simulink model "v2022_Modello_SITL_AENEA_2020b"  (R2020b)
settings: Solver=ode4  StartTime=0.0  StopTime=500  FixedStep=0.01  RelTol=1e-3
values from neighbouring files (symbols this model uses):
  attuatore_Amax = 20*(pi/180)    (= 0.349065850399)    [v2021_10_27_avvioSITL.m]
  attuatore_Emax = 25*(pi/180)    (= 0.436332312999)    [v2021_10_27_avvioSITL.m]
  attuatore_Rmax = 25*(pi/180)    (= 0.436332312999)    [v2021_10_27_avvioSITL.m]
  beta_phi = 1/10.5600    (= 0.094696969697)    [Load_modello_sensori.m]
  beta_psi = 1/170    (= 0.00588235294118)    [Load_modello_sensori.m]
  beta_theta = 1/10.5000    (= 0.0952380952381)    [Load_modello_sensori.m]
  CldR = KCldR(1)*180/pi    [Timone.m]
  CndR = KCndR(1)*180/pi    [Timone.m]
  CYdR = -KCYdR(1)*180/pi    [Timone.m]
  delay_ahrs = 0    [Load_modello_sensori.m]
  delay_bmp = 0    [Load_modello_sensori.m]
  delay_gps = 0    [Load_modello_sensori.m]
  deltaAtrim = 0    [v2021_10_27_avvioSITL.m]
  deltaEtrim = (Cm0*CL_alpharad+Cm_alpharad*CLtrim)/(CL_alpharad*CmdE)    [calcoloDatiIniziali.m]    (also in v2021_10_27_avvioSITL.m = 0)
  deltaRtrim = 0    [v2021_10_27_avvioSITL.m]
  deltaTtrim = 0.1    [v2021_10_27_avvioSITL.m]
  HINI = -State0.Pos0(3)    [v2021_10_27_avvioSITL.m]
  Ingaggio_AP = input("inserire 1 se si vuole ingaggiare l' AP, 0 altrimenti: ")    [v2021_10_27_avvioSITL.m]
  J_vec = [0 0.03 0.06 0.09 0.11 0.14 0.17 0.2 0.23 0.26 0.28 0.31 ... (30 elements, 30x1)]    [PropLUT.mat]
  latitudineINI = 42.07278258649732*pi/180    (= 0.73430858161)    [v2021_10_27_avvioSITL.m]
  longitudineINI = 12.615743929793046*pi/180    (= 0.220186269163)    [v2021_10_27_avvioSITL.m]
  mean_ax = 0*0.0392    (= 0)    [Load_modello_sensori.m]
  mean_ay = -0*0.0598    (= 0)    [Load_modello_sensori.m]
  mean_az = 0*0.0384    (= 0)    [Load_modello_sensori.m]
  mean_p = 0*1.5184e-06    (= 0)    [Load_modello_sensori.m]
  mean_q = 0*2.9671e-05    (= 0)    [Load_modello_sensori.m]
  mean_r = 0*5.4105e-05    (= 0)    [Load_modello_sensori.m]
  P_ref = 1.0074e+05    (= 100740)    [Load_modello_sensori.m]
  PWM_Aileron = rad2deg(deltaAtrim)*9+1503    [v2021_10_27_avvioSITL.m]
  PWM_Elevator = rad2deg(deltaEtrim)*(447/50)+(3007/2)    [v2021_10_27_avvioSITL.m]
  PWM_Rudder = rad2deg(deltaRtrim)*(447/50)+(3007/2)    [v2021_10_27_avvioSITL.m]
  PWM_Throttle = (deltaTtrim)*800+1100    (= 1180)    [v2021_10_27_avvioSITL.m]
  seed_ahrs = randi([0 2000],1,1)    [Load_modello_sensori.m]
  seed_baro = randi([0 2000],1,1)    [Load_modello_sensori.m]
  seed_gps = randi([0 2000],1,1)    [Load_modello_sensori.m]
  sensori_FreqCampionamento_pitot = 0.02    [v2021_10_27_avvioSITL.m]
  sensori_RumoreSampleTime = 0.02    [v2021_10_27_avvioSITL.m]
  sensori_varianza = 0.0000    (= 0)    [v2021_10_27_avvioSITL.m]
  Std_con_lat = 7.501025208540287e-07    (= 7.50102520854e-07)    [Load_modello_sensori.m]
  Std_con_long = 5.101110498551838e-06    (= 5.10111049855e-06)    [Load_modello_sensori.m]
  Std_vel = 0.05    [Load_modello_sensori.m]
  T0_ref = 25    [Load_modello_sensori.m]
  Ta_lat = 10^2    (= 100)    [Load_modello_sensori.m]
  Ta_long = 10^2    (= 100)    [Load_modello_sensori.m]
  Ts_ahrs = 0.02    [Load_modello_sensori.m]
  Ts_bmp = 0.02    [Load_modello_sensori.m]
  Ts_gps = 0.1    [Load_modello_sensori.m]
  tsamp = 0.02    [v2021_10_27_avvioSITL.m]
  Var_heading = 0.0025    [Load_modello_sensori.m]
  Var_heading_static = 0.0625    [Load_modello_sensori.m]
  Var_V_hor = 0.1    [Load_modello_sensori.m]
  Var_V_hor_static = 0.04    [Load_modello_sensori.m]
  White_ax = 1.486e-04    (= 0.0001486)    [Load_modello_sensori.m]
  White_ay = 9.403e-05    [Load_modello_sensori.m]
  White_az = 1.648e-04    (= 0.0001648)    [Load_modello_sensori.m]
  White_gm_phi = 3.2740e-05    (= 3.274e-05)    [Load_modello_sensori.m]
  White_gm_psi = 2.9162e-04    (= 0.00029162)    [Load_modello_sensori.m]
  White_gm_theta = 2.4704e-05    [Load_modello_sensori.m]
  White_p = 2.934e-05    [Load_modello_sensori.m]
  White_pressione = 10.18    [Load_modello_sensori.m]
  White_r = 3.258e-05    [Load_modello_sensori.m]
  WP_AL = [     0 20 0 0 41.807822 12.589274 3 ... (first row only)    [v2021_10_27_avvioSITL.m]
  WP_CV = input('simulare waypoint provenienti da CV 1, 0 altrimenti')    [v2021_10_27_avvioSITL.m]
  WP_db_info = [6 1 0 0 1 1;             6 2 0 0 0 1;              6 3 0 0 0 1;              6 4 0 0 0 1 ... (first row only)    [v2021_10_27_avvioSITL.m]
  WP_db_info_CV = [6 1 0 0 1 1;             6 2 0 0 0 1;              6 3 0 0 0 0;              6 4 0 0 0 0 ... (first row only)    [v2021_10_27_avvioSITL.m]
  WP_db_param = [ 0 0 23 0 42.067940318394974 12.61119490312005 40 ... (first row only)    [v2021_10_27_avvioSITL.m]
  WP_db_param_CV = [ 0 0 23 0 42.05047960115445 12.622867877224342 40 ... (first row only)    [v2021_10_27_avvioSITL.m]
  Zpista = 0    [v2021_10_27_avvioSITL.m]
undefined symbols (not defined in the file or in its folder): alphavec_rad, b, betavec_rad, c, cbar, CD0, CldA, CLdE, Clp, CLq, Clr, CmdE, Cmq, CndA, Cnp, Cnr, CYdA, CYp, CYr, Dprop, Earth, F, g, h_home, Jeng, Jprop, matricepolinomi, MIL, rACtG, rACwG, rAHRSG, Receive, rho, rLEG, rmglG, rmgrG, rngG, rNPG, rPG, Rprop, S, Send, State0, V_cruise, W, WGS84, Zeng
libraries: simulink_extras x27, aerolibfltsims x5, simulink x3, aerolibwind2 x3, aerolibasang x2, shared6dof x1, slpidlib x1, aerolibatmos2 x1, aerolibanimutils x1
(part 2 of 3)

== system v2022_Modello_SITL_AENEA_2020b/Sensori/Sensore di pressione differenziale ==
  note: Modello di errore del sensore di pressione differenziale aggiunto da Emanuele D'Alessio ed Emanuele Perfetti in data 12/03/2022. Ci si è basati sulla tesi di Di Giulio.
  In1 : Inport
  Constant : Constant  Value=2
  Constant1 : Constant  Value=rho
  Divide : Product  Inputs=*/
  Product : Product
  Rate Transition23 : RateTransition  OutPortSampleTime=0.02
  Sqrt : Sqrt  SaturateOnIntegerOverflow=on
  Sum3 : Sum  Inputs=++|
  White Noise1 : RandomNumber  DisableCoverage=on  Variance=3.9744  Seed=[23341]  SampleTime=sensori_RumoreSampleTime
  Zero-Order Hold19 : ZeroOrderHold  SampleTime=sensori_FreqCampionamento_pitot
  Out1 : Outport
  wires:
  White Noise1/1 -> Sum3/1
  Zero-Order Hold19/1 -> Rate Transition23/1  "deltaP"
  In1/1 -> Sum3/2
  Sum3/1 -> Zero-Order Hold19/1  "deltaP"
  Rate Transition23/1 -> Product/2  "deltaP"
  Constant/1 -> Product/1
  Product/1 -> Divide/1
  Constant1/1 -> Divide/2
  Divide/1 -> Sqrt/1
  Sqrt/1 -> Out1/1  "Ias"

== system v2022_Modello_SITL_AENEA_2020b/Sensori/int1 ==
  In1 : Inport
  "INT16 " : Subsystem
  Out1 : Outport  VectorParamsAs1DForOutWhenUnconnected=off
  wires:
  In1/1 -> "INT16 "/1(<u>)
  "INT16 "/1(Out1) -> Out1/1

== system v2022_Modello_SITL_AENEA_2020b/Sensori/int16 ==
  In1 : Inport
  "INT16 " : Subsystem
  Out1 : Outport  VectorParamsAs1DForOutWhenUnconnected=off
  wires:
  "INT16 "/1(Out1) -> Out1/1
  In1/1 -> "INT16 "/1(<u>)

== system v2022_Modello_SITL_AENEA_2020b/Sensori/int16_rad  ==
  In1 : Inport
  Degrees to Radians : simulink_extras/Transformations/Degrees to Radians
  "INT16 " : Subsystem
  Radians to Degrees : simulink_extras/Transformations/Radians to Degrees
  Out1 : Outport  VectorParamsAs1DForOutWhenUnconnected=off
  wires:
  In1/1 -> Radians to Degrees/1
  "INT16 "/1(Out1) -> Degrees to Radians/1
  Degrees to Radians/1 -> Out1/1
  Radians to Degrees/1 -> "INT16 "/1(<u>)

== system v2022_Modello_SITL_AENEA_2020b/Sensori/int16_rad 1 ==
  In1 : Inport
  Degrees to Radians : simulink_extras/Transformations/Degrees to Radians
  "INT16 " : Subsystem
  Radians to Degrees : simulink_extras/Transformations/Radians to Degrees
  Out1 : Outport  VectorParamsAs1DForOutWhenUnconnected=off
  wires:
  Degrees to Radians/1 -> Out1/1
  In1/1 -> Radians to Degrees/1
  Radians to Degrees/1 -> "INT16 "/1(<u>)
  "INT16 "/1(Out1) -> Degrees to Radians/1

== system v2022_Modello_SITL_AENEA_2020b/Sensori/int16_rad 2 ==
  In1 : Inport
  Degrees to Radians : simulink_extras/Transformations/Degrees to Radians
  "INT16 " : Subsystem
  Radians to Degrees : simulink_extras/Transformations/Radians to Degrees
  Out1 : Outport  VectorParamsAs1DForOutWhenUnconnected=off
  wires:
  In1/1 -> Radians to Degrees/1
  "INT16 "/1(Out1) -> Degrees to Radians/1
  Radians to Degrees/1 -> "INT16 "/1(<u>)
  Degrees to Radians/1 -> Out1/1

== system v2022_Modello_SITL_AENEA_2020b/Sensori/int16_rad 3 ==
  In1 : Inport
  Degrees to Radians : simulink_extras/Transformations/Degrees to Radians
  "INT16 " : Subsystem
  Radians to Degrees : simulink_extras/Transformations/Radians to Degrees
  Out1 : Outport  VectorParamsAs1DForOutWhenUnconnected=off
  wires:
  "INT16 "/1(Out1) -> Degrees to Radians/1
  In1/1 -> Radians to Degrees/1
  Radians to Degrees/1 -> "INT16 "/1(<u>)
  Degrees to Radians/1 -> Out1/1

== system v2022_Modello_SITL_AENEA_2020b/Sensori/int16_rad 4 ==
  In1 : Inport
  Degrees to Radians : simulink_extras/Transformations/Degrees to Radians
  "INT16 " : Subsystem
  Radians to Degrees : simulink_extras/Transformations/Radians to Degrees
  Out1 : Outport  VectorParamsAs1DForOutWhenUnconnected=off
  wires:
  In1/1 -> Radians to Degrees/1
  "INT16 "/1(Out1) -> Degrees to Radians/1
  Radians to Degrees/1 -> "INT16 "/1(<u>)
  Degrees to Radians/1 -> Out1/1

== system v2022_Modello_SITL_AENEA_2020b/Sensori/int16_rad 5 ==
  In1 : Inport
  Degrees to Radians : simulink_extras/Transformations/Degrees to Radians
  "INT16 " : Subsystem
  Radians to Degrees : simulink_extras/Transformations/Radians to Degrees
  Out1 : Outport  VectorParamsAs1DForOutWhenUnconnected=off
  wires:
  "INT16 "/1(Out1) -> Degrees to Radians/1
  In1/1 -> Radians to Degrees/1
  Radians to Degrees/1 -> "INT16 "/1(<u>)
  Degrees to Radians/1 -> Out1/1

== system v2022_Modello_SITL_AENEA_2020b/Sensori/int2 ==
  In1 : Inport
  "INT16 " : Subsystem
  Out1 : Outport  VectorParamsAs1DForOutWhenUnconnected=off
  wires:
  "INT16 "/1(Out1) -> Out1/1
  In1/1 -> "INT16 "/1(<u>)

== system v2022_Modello_SITL_AENEA_2020b/Sensori/single 1 ==
  <u> : Inport
  Data Type Conversion1 : DataTypeConversion  OutDataTypeStr=double  LockScale=on
  Data Type Conversion2 : DataTypeConversion  OutDataTypeStr=single  LockScale=on
  Degrees to Radians : simulink_extras/Transformations/Degrees to Radians
  Radians to Degrees : simulink_extras/Transformations/Radians to Degrees
  Out1 : Outport  VectorParamsAs1DForOutWhenUnconnected=off
  wires:
  Data Type Conversion1/1 -> Degrees to Radians/1
  <u>/1 -> Radians to Degrees/1
  Data Type Conversion2/1 -> Data Type Conversion1/1
  Radians to Degrees/1 -> Data Type Conversion2/1
  Degrees to Radians/1 -> Out1/1

== system v2022_Modello_SITL_AENEA_2020b/Sensori/single 3 ==
  <u> : Inport
  Data Type Conversion1 : DataTypeConversion  OutDataTypeStr=double  LockScale=on
  Data Type Conversion2 : DataTypeConversion  OutDataTypeStr=single  LockScale=on
  Out1 : Outport  VectorParamsAs1DForOutWhenUnconnected=off
  wires:
  Data Type Conversion1/1 -> Out1/1
  <u>/1 -> Data Type Conversion2/1
  Data Type Conversion2/1 -> Data Type Conversion1/1

== system v2022_Modello_SITL_AENEA_2020b/Sensori/single 4 ==
  <u> : Inport
  Data Type Conversion1 : DataTypeConversion  OutDataTypeStr=double  LockScale=on
  Data Type Conversion2 : DataTypeConversion  OutDataTypeStr=single  LockScale=on
  Degrees to Radians : simulink_extras/Transformations/Degrees to Radians
  Radians to Degrees : simulink_extras/Transformations/Radians to Degrees
  Out1 : Outport  VectorParamsAs1DForOutWhenUnconnected=off
  wires:
  Data Type Conversion2/1 -> Data Type Conversion1/1
  <u>/1 -> Radians to Degrees/1
  Data Type Conversion1/1 -> Degrees to Radians/1
  Radians to Degrees/1 -> Data Type Conversion2/1
  Degrees to Radians/1 -> Out1/1

== system v2022_Modello_SITL_AENEA_2020b/AENEA /AENEA II_SITL1/Forze aerodinamiche ==
  ωb : Inport
  qbar : Inport  Port=2
  Vect_Comandi : Inport  Port=3
  Vect_Costanti : Inport  Port=4
  "Vbpolare " : Inport  Port=5
  Bus Creator : BusCreator  Inputs=3
  Bus Selector : BusSelector  OutputSignals=α,β
  Bus Selector1 : BusSelector  OutputSignals=Coef_Geometrici.S
  Demux : Demux  Outputs=3
  Forze assi vento/q : Subsystem
  MATLAB Function : MATLAB Function  TreatAsAtomicUnit=on
  Matrix Multiply : Product  Multiplication=Matrix(*)
  Momenti /press din : Subsystem
  Product : Product  Inputs=3
  Product2 : Product
  FA_B : Outport  VectorParamsAs1DForOutWhenUnconnected=off
  MA_B : Outport  Port=2  VectorParamsAs1DForOutWhenUnconnected=off
  CL : Outport  Port=3  VectorParamsAs1DForOutWhenUnconnected=off
  wires:
  Product2/1 -> MA_B/1
  Product/1 -> FA_B/1
  qbar/1 -> Product/3, Product2/1
  ωb/1 -> Demux/1
  Demux/1 -> Bus Creator/1  "p"
  Demux/2 -> Bus Creator/2  "q"
  Demux/3 -> Bus Creator/3  "r"
  Bus Selector/1 -> MATLAB Function/1(alpha)  "<α>"
  Bus Selector/2 -> MATLAB Function/2(beta)  "<β>"
  MATLAB Function/1(Lbw) -> Matrix Multiply/1
  Matrix Multiply/1 -> Product/2  "FA_B/q"
  Momenti /press din/1(MA_B/q) -> Product2/2
  Forze assi vento/q/1(FA_W/q) -> Matrix Multiply/2
  Vect_Comandi/1 -> Forze assi vento/q/1(Vect_Comandi), Momenti /press din/1(Vect_Comandi)
  "Vbpolare "/1 -> Bus Selector/1, Forze assi vento/q/3("Vbpolare "), Momenti /press din/3("Vbpolare ")
  Bus Creator/1 -> Momenti /press din/4(ωb), Forze assi vento/q/4(ωb)  "ωb"
  Vect_Costanti/1 -> Bus Selector1/1, Forze assi vento/q/2(Vect_Costanti), Momenti /press din/2(Vect_Costanti)
  Bus Selector1/1 -> Product/1  "<S>"
  Forze assi vento/q/2(CL) -> CL/1

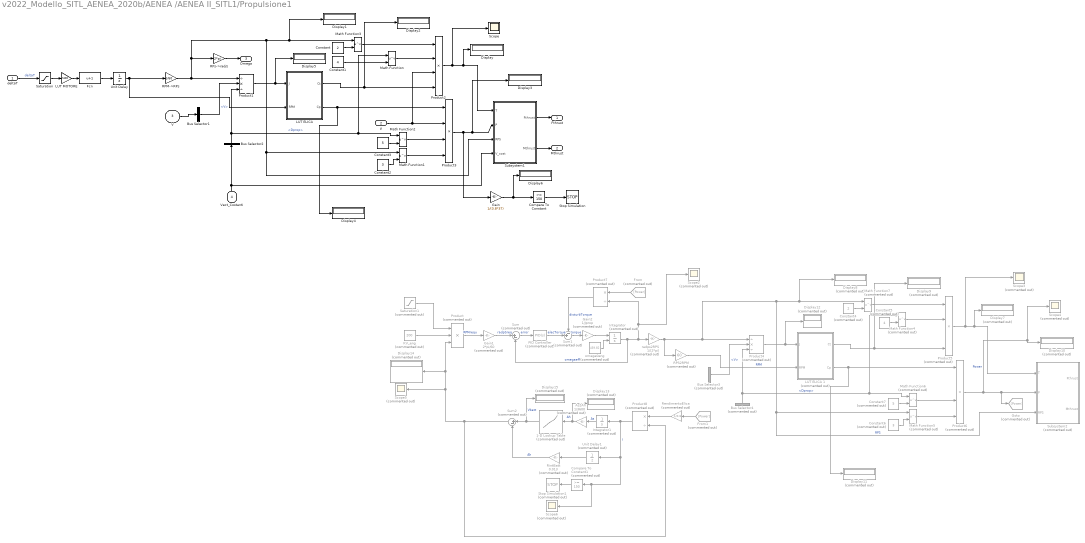
== system v2022_Modello_SITL_AENEA_2020b/AENEA /AENEA II_SITL1/Propulsione1 ==
  "deltaT " : Inport
  ρ : Inport  Port=2
  V : Inport  Port=3
  Vect_Costanti : Inport  Port=4
  1-D Lookup Table : Lookup_n-D  Commented=on  NumberOfTableDimensions=1  BreakpointsForDimension1=[0,5,5.2]  Table=[42,34,0]  InternalRulePriority=Speed  RndMeth=Simplest  InputSameDT=on
  As2Ah : Gain  Commented=on  Gain=1/3600
  Bus Selector1 : BusSelector  OutputSignals=V
  Bus Selector2 : BusSelector  OutputSignals=Coef_Geometrici.Dprop
  Bus Selector3 : BusSelector  Commented=on  OutputSignals=V
  Bus Selector4 : BusSelector  Commented=on  OutputSignals=Coef_Geometrici.Dprop
  Compare To Constant : simulink/Logic and Bit Operations/Compare To Constant  relop=>=  const=150  OutDataTypeStr=boolean
  Compare To Constant1 : simulink/Logic and Bit Operations/Compare To Constant  Commented=on  relop=>=  const=150  OutDataTypeStr=boolean
  Constant : Constant  Value=2
  Constant1 : Constant  Value=4
  Constant2 : Constant  Value=3
  Constant3 : Constant  Value=5
  Constant4 : Constant  Commented=on  Value=2
  Constant5 : Constant  Commented=on  Value=4
  Constant6 : Constant  Commented=on  Value=3
  Constant7 : Constant  Commented=on  Value=5
  Display{,1..6} (7 alike) : Display
  Display{7..15} (9 alike) : Display  Commented=on
  Fcn : Fcn  Expr=u+1
  From : From  Commented=on  GotoTag=Power
  From1 : From  Commented=on  GotoTag=Power
  Gain : Gain  Gain=1/(0.8*37)
  Gain1 : Gain  Commented=on  Gain=2*pi/60
  Gain2 : Gain  Commented=on  Gain=1/Jprop
  Goto : Goto  Commented=on  GotoTag=Power
  Integrator : Integrator  Commented=on  InitialConditionSource=external
  Integrator1 : Integrator  Commented=on
  "KV_eng " : Constant  Commented=on  Value=200
  "LUT ELICA " : Subsystem
  LUT ELICA 1 : Subsystem  Commented=on
  LUT MOTORE : Gain  Gain=7400
  Math Function{,1..3} (4 alike) : Math  Operator=pow  SignedPower=on  SaturateOnIntegerOverflow=on
  Math Function{4..7} (4 alike) : Math  Commented=on  Operator=pow  SignedPower=on  SaturateOnIntegerOverflow=on
  PID Controller : slpidlib/PID Controller  Commented=on  Controller=PID  Form=Parallel  TimeDomain=Continuous-time  UseExternalTs=off  SampleTime=-1  IntegratorMethod=Forward Euler  FilterMethod=Forward Euler  ControllerParametersSource=internal  P=0.7  I=0.1  D=0  UseFilter=on  N=100  TunerSelectOption=Frequency Response Based  InitialConditionSource=internal  InitialConditionForIntegrator=0  InitialConditionForFilter=0  DifferentiatorICPrevScaledInput=0  ExternalReset=none  TrackingMode=off  Kt=1  LimitOutput=off  SatLimitsSource=internal  UpperSaturationLimit=inf  LowerSaturationLimit=-inf  LinearizeAsGain=on  AntiWindupMode=none  Kb=1  POutMin=[]  POutMax=[]  IOutMin=[]  IOutMax=[]  DOutMin=[]  DOutMax=[]  NOutMin=[]  NOutMax=[]  SumOutMin=[]  SumOutMax=[]  SaturationOutMin=[]  SaturationOutMax=[]  PParamMin=[]  PParamMax=[]  IParamMin=[]  IParamMax=[]  DParamMin=[]  DParamMax=[]  NParamMin=[]  NParamMax=[]  KbParamMin=[]  KbParamMax=[]  KtParamMin=[]  KtParamMax=[]  KbOutMin=[]  KbOutMax=[]  KtOutMin=[]  KtOutMax=[]  IntegratorOutMin=[]  IntegratorOutMax=[]  FilterOutMin=[]  FilterOutMax=[]  SumI1OutMin=[]  SumI1OutMax=[]  SumI2OutMin=[]  SumI2OutMax=[]  SumI3OutMin=[]  SumI3OutMax=[]  SumI4OutMin=[]  SumI4OutMax=[]  SumDOutMin=[]  SumDOutMax=[]  DifferentiatorOutMin=[]  DifferentiatorOutMax=[]  FilterDiffOutCoefMin=[]  FilterDiffOutCoefMax=[]  ReciprocalOutMin=[]  ReciprocalOutMax=[]  SumDenOutMin=[]  SumDenOutMax=[]  SumNumOutMin=[]  SumNumOutMax=[]  DivideOutMin=[]  DivideOutMax=[]  UdiffTsProdOutMin=[]  UdiffTsProdOutMax=[]  NTsProdOutMin=[]  NTsProdOutMax=[]  UintegralTsProdOutMin=[]  UintegralTsProdOutMax=[]  UngainTsProdOutMin=[]  UngainTsProdOutMax=[]  IntegratorContinuousStateAttributes=''  IntegratorStateMustResolveToSignalObject=off  IntegratorRTWStateStorageClass=Auto  FilterContinuousStateAttributes=''  FilterStateMustResolveToSignalObject=off  FilterRTWStateStorageClass=Auto  ParallelPVariant=InternalParameters  IdealPVariant=Disabled  IVariant=InternalParameters  DVariant=InternalParameters  IntegratorVariant=Continuous  SatVariant=Disabled  AWVariant=Passthrough  PCopyVariant=Disabled  TRVariant=Disabled  FdbkBlocksVariant=Forward  IdealPFdbkVariant=Disabled  SatFdbkVariant=Disabled  DerivativeFilterVariant=ContFilter  NVariant=InternalParameters  NCopyVariant=Disabled  FilterICVariant=InternalICsFilter  IntegratorICVariant=InternalICs  ExternalResetVariant=Disabled  TRSumVariant=Passthrough  SumFdbkVariant=Disabled  SumVariant=Sum_PID  TsampFilterVariant=InternalTs  TsampNgainVariant=Passthrough  TsampIntegralVariant=Passthrough  ExternalSaturationOutDataTypeStr=Inherit: Same as second input
  Product : Product  Commented=on  Inputs=3
  Product1 : Product  Inputs=/*/
  Product2 : Product  Inputs=****
  Product3 : Product  Inputs=****
  Product4 : Product  Commented=on  Inputs=/*/
  Product5 : Product  Commented=on  Inputs=****
  Product6 : Product  Commented=on  Inputs=****
  Product7 : Product  Commented=on  Inputs=*/
  Product8 : Product  Commented=on  Inputs=*/
  RPM->RPs : Gain  Gain=1/60
  "RPS2RPM  " : Gain  Commented=on  Gain=60
  RPs->rad/s : Gain  Gain=2*pi
  "RendimentoElica " : Gain  Commented=on  Gain=1/0.8
  "RintBatt " : Gain  Commented=on  Gain=0.013
  Saturation : Saturate  UpperLimit=1  LowerLimit=0
  Saturation1 : Saturate  Commented=on  UpperLimit=1  LowerLimit=0
  Scope : Scope
  Scope{2..6} (5 alike) : Scope  Commented=on
  Stop Simulation : Stop
  Stop Simulation1 : Stop  Commented=on
  Subsystem1 : Subsystem
  Subsystem2 : Subsystem  Commented=on
  Sum : Sum  Commented=on  Inputs=|+-
  Sum1 : Sum  Commented=on  Inputs=-+|
  Sum2 : Sum  Commented=on  Inputs=|+-
  Unit Delay : UnitDelay  InitialCondition=deltaTtrim*7400  SampleTime=-1  HasFrameUpgradeWarning=on
  Unit Delay1 : UnitDelay  Commented=on  SampleTime=0.01  HasFrameUpgradeWarning=on
  omega0eng : Constant  Commented=on  Value=439.82
  radps2RPS : Gain  Commented=on  Gain=1/(2*pi)
  "Fthrust " : Outport  VectorParamsAs1DForOutWhenUnconnected=off
  Mthrust : Outport  Port=2  VectorParamsAs1DForOutWhenUnconnected=off
  Omega : Outport  Port=3
  wires:
  Vect_Costanti/1 -> Subsystem1/4(V_cost), Bus Selector2/1
  "deltaT "/1 -> Saturation/1  "deltaT"
  V/1 -> Bus Selector1/1
  Bus Selector1/1 -> Product1/2  "<V>"
  Bus Selector2/1 -> Math Function2/1, Math Function/1, Product1/3  "<Dprop>"
  Product1/1 -> "LUT ELICA "/1(J), Display5/1
  ρ/1 -> Product2/3, Product3/2
  "LUT ELICA "/2(Cp) -> Display4/1, Product3/1
  "LUT ELICA "/1(Ct) -> Display2/1, Product2/4
  Math Function3/1 -> Product2/1
  Math Function/1 -> Product2/2
  Constant/1 -> Math Function3/2
  Constant1/1 -> Math Function/2
  Math Function2/1 -> Product3/3
  Constant3/1 -> Math Function2/2
  Constant2/1 -> Math Function1/2
  Math Function1/1 -> Product3/4
  Product2/1 -> Scope/1, Display/1, Subsystem1/1(T)
  Subsystem1/1(Fthrust) -> "Fthrust "/1
  Subsystem1/2("Mthrust ") -> Mthrust/1
  Product3/1 -> Gain/1, Display3/1, Subsystem1/2(P)
  Gain/1 -> Display6/1, Compare To Constant/1
  Compare To Constant/1 -> Stop Simulation/1
  RPs->rad/s/1 -> Omega/1
  RPM->RPs/1 -> RPs->rad/s/1, Subsystem1/3(RPS), Math Function1/1, Display1/1, Math Function3/1, Product1/1
  Saturation/1 -> LUT MOTORE/1
  Unit Delay/1 -> "LUT ELICA "/2(RPM), RPM->RPs/1
  LUT MOTORE/1 -> Fcn/1
  Fcn/1 -> Unit Delay/1
  omega0eng/1 -> Integrator/2
  Saturation1/1 -> Product/1
  Product/1 -> Gain1/1  "RPMrequ"
  From1/1 -> "RendimentoElica "/1
  Product7/1 -> Sum1/1  "disturbTorque"
  "RendimentoElica "/1 -> Product8/1
  "RintBatt "/1 -> Sum2/2  "Ah"
  Unit Delay1/1 -> "RintBatt "/1
  Sum2/1 -> Product8/2, Scope5/1, Display14/1, Product/3
  LUT ELICA 1/1(Ct) -> Display9/1, Product5/4
  Product8/1 -> Scope6/1, Compare To Constant1/1, Unit Delay1/1, Integrator1/1  "I"
  Bus Selector4/1 -> Math Function6/1, Math Function4/1, Product4/3  "<Dprop>"
  PID Controller/1 -> Sum1/2  "elecTorque"
  Integrator/1 -> Sum/2, Scope2/1, Product7/2, radps2RPS/1  "omegaeff"
  1-D Lookup Table/1 -> Display15/1, Sum2/1  "Vbatt"
  "KV_eng "/1 -> Product/2
  Math Function6/1 -> Product6/3
  Gain1/1 -> Sum/1  "radpSreq"
  Product6/1 -> Scope4/1, Display10/1, Goto/1, Subsystem2/2(P)  "Power"
  Sum1/1 -> Gain2/1  "torque"
  Compare To Constant1/1 -> Stop Simulation1/1
  LUT ELICA 1/2(Cp) -> Display11/1, Product6/1
  Integrator1/1 -> As2Ah/1  "As"
  Math Function7/1 -> Product5/1
  Sum/1 -> PID Controller/1  "error"
  As2Ah/1 -> Display13/1, 1-D Lookup Table/1  "Ah"
  Product5/1 -> Scope3/1, Display7/1, Subsystem2/1(T)
  Math Function5/1 -> Product6/4
  "RPS2RPM  "/1 -> LUT ELICA 1/2(RPM)  "RPM"
  From/1 -> Product7/1
  Math Function4/1 -> Product5/2
  Constant4/1 -> Math Function7/2
  Constant6/1 -> Math Function5/2
  Constant7/1 -> Math Function6/2
  Product4/1 -> Display12/1, LUT ELICA 1/1(J)
  radps2RPS/1 -> "RPS2RPM  "/1, Subsystem2/3(RPS), Math Function5/1, Display8/1, Math Function7/1, Product4/1  "RPS"
  Gain2/1 -> Integrator/1
  Bus Selector3/1 -> Product4/2  "<V>"
  Constant5/1 -> Math Function4/2

== system v2022_Modello_SITL_AENEA_2020b/AENEA /AENEA II_SITL1/Subsystem ==
  xE : Inport
  Φvect : Inport  Port=2
  Vb : Inport  Port=3
  ω_b : Inport  Port=4
  Bus Creator1 : BusCreator  Inputs=4
  Bus Creator{3..4,8..9} (4 alike) : BusCreator  Inputs=3
  Demux{1..2,6..7} (4 alike) : Demux  Outputs=3
  Scope : Scope
  "Xstato " : Outport  VectorParamsAs1DForOutWhenUnconnected=off
  wires:
  Demux2/3 -> Bus Creator4/3  "r"
  Bus Creator4/1 -> Bus Creator1/3  "ωvect"
  Φvect/1 -> Demux6/1
  Vb/1 -> Demux7/1
  Bus Creator8/1 -> Bus Creator1/2  "PhiThetaPsi"
  Demux1/3 -> Bus Creator3/3  "h"
  Demux2/2 -> Bus Creator4/2  "q"
  Demux2/1 -> Bus Creator4/1  "p"
  Bus Creator3/1 -> Bus Creator1/4  "xyz"
  ω_b/1 -> Demux2/1
  Demux6/3 -> Scope/1, Bus Creator8/3  "Psi"
  Demux6/1 -> Bus Creator8/1  "Phi"
  Demux1/1 -> Bus Creator3/1  "x"
  Demux7/1 -> Bus Creator9/1  "u"
  Demux7/3 -> Bus Creator9/3  "w"
  Bus Creator9/1 -> Bus Creator1/1  "uvw"
  Demux1/2 -> Bus Creator3/2  "y"
  Demux7/2 -> Bus Creator9/2  "v"
  Demux6/2 -> Bus Creator8/2  "Theta"
  Bus Creator1/1 -> "Xstato "/1  "Xstato"
  xE/1 -> Demux1/1

== system v2022_Modello_SITL_AENEA_2020b/AENEA /AENEA II_SITL1/Subsystem1 ==
  omegapunto : Inport
  V : Inport  Port=2
  Abb : Inport  Port=3
  "PhiThetaPsipunto " : Inport  Port=4
  Bus Creator{5,7,10..11} (4 alike) : BusCreator  Inputs=3
  Bus Creator6 : BusCreator  Inputs=4
  Demux{3..4,8..9} (4 alike) : Demux  Outputs=3
  Xpunto : Outport  VectorParamsAs1DForOutWhenUnconnected=off
  wires:
  Demux4/3 -> Bus Creator7/3  "wpunto"
  Demux3/1 -> Bus Creator5/1  "ppunto"
  Demux4/2 -> Bus Creator7/2  "vpunto"
  Demux8/2 -> Bus Creator10/2  "Thetapunto"
  Bus Creator10/1 -> Bus Creator6/2  "EulerAnglespunto"
  Demux3/2 -> Bus Creator5/2  "qpunto"
  Demux4/1 -> Bus Creator7/1  "upunto"
  V/1 -> Demux9/1
  Demux8/1 -> Bus Creator10/1  "Phipunto"
  Bus Creator11/1 -> Bus Creator6/4  "xyzpunto"
  Demux8/3 -> Bus Creator10/3  "Psipunto"
  Demux3/3 -> Bus Creator5/3  "rpunto"
  Demux9/2 -> Bus Creator11/2  "Yepunto"
  Bus Creator7/1 -> Bus Creator6/1  "Vbpunto"
  Bus Creator5/1 -> Bus Creator6/3  "ωpunto"
  Demux9/1 -> Bus Creator11/1  "Xepunto"
  Demux9/3 -> Bus Creator11/3  "Zepunto"
  "PhiThetaPsipunto "/1 -> Demux8/1
  omegapunto/1 -> Demux3/1
  Abb/1 -> Demux4/1
  Bus Creator6/1 -> Xpunto/1

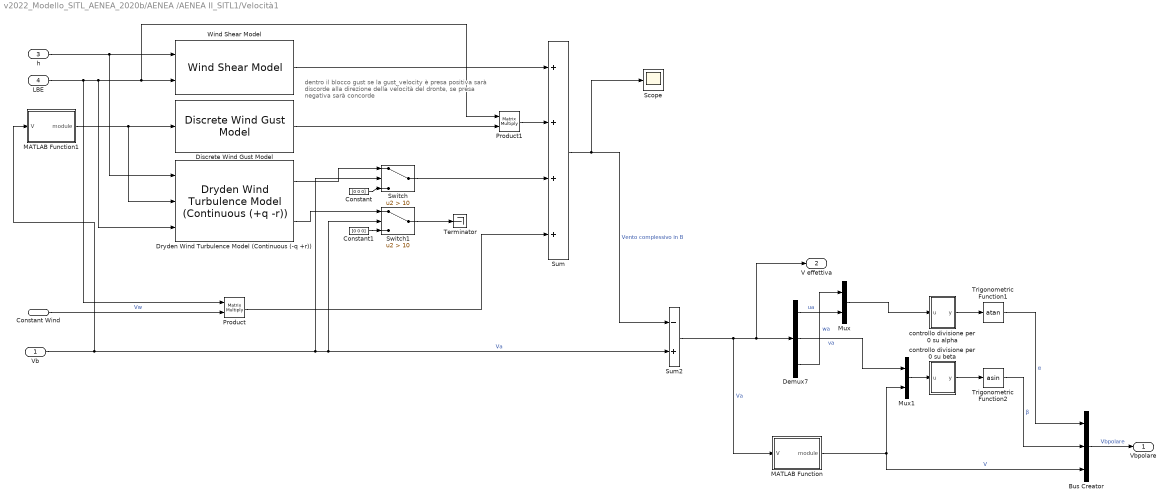
== system v2022_Modello_SITL_AENEA_2020b/AENEA /AENEA II_SITL1/Velocità1 ==
  note: dentro il blocco gust se la gust_velocity è presa positiva sarà discorde alla direzione della velocità del dronte, se presa negativa sarà concorde
  Vb : Inport
  Constant Wind : Inport  Port=2
  h : Inport  Port=3
  LBE : Inport  Port=4
  Bus Creator : BusCreator  Inputs=3
  Constant : Constant  Value=[0 0 0]
  Constant1 : Constant  Value=[0 0 0]
  Demux7 : Demux  Outputs=3
  Discrete Wind Gust Model : aerolibwind2/Discrete Wind Gust Model  units=Metric (MKS)  Gx=on  Gy=on  Gz=on  t_0=0  d_m=[120 120 80]  v_m=[0 0 0]
  Dryden Wind Turbulence Model (Continuous (-q +r)) : aerolibwind2/Dryden Wind Turbulence Model  (Continuous (+q -r))  units=Metric (MKS)  spec=MIL-F-8785C  model=Continuous Dryden (-q +r)  W20=0  Wdeg=180  TurbProb=10^-4  L_high=533.4  Wingspan=2.6  ts=0.01  Seed=[23341 23342 23343 23344]  T_on=on
  MATLAB Function : MATLAB Function  TreatAsAtomicUnit=on
  MATLAB Function1 : MATLAB Function  TreatAsAtomicUnit=on
  Mux : Mux  Inputs=2
  Mux1 : Mux  Inputs=2
  Product : Product  Multiplication=Matrix(*)
  Product1 : Product  Multiplication=Matrix(*)
  Scope : Scope
  Sum : Sum  Inputs=4
  Sum2 : Sum  Inputs=-+
  Switch : Switch  Criteria=u2 > Threshold  Threshold=10
  Switch1 : Switch  Criteria=u2 > Threshold  Threshold=10
  Terminator : Terminator
  Trigonometric Function1 : Trigonometry  Operator=atan
  Trigonometric Function2 : Trigonometry  Operator=asin
  Wind Shear Model : aerolibwind2/Wind Shear Model  units=Metric (MKS)  phase=Category C - Terminal Flight Phase  W_20=0  Wdeg=180
  controllo divisione per 0 su alpha : MATLAB Function  TreatAsAtomicUnit=on
  controllo divisione per 0 su beta : MATLAB Function  TreatAsAtomicUnit=on
  Vbpolare : Outport  VectorParamsAs1DForOutWhenUnconnected=off
  "V effettiva " : Outport  Port=2  VectorParamsAs1DForOutWhenUnconnected=off
  wires:
  Bus Creator/1 -> Vbpolare/1  "Vbpolare"
  Trigonometric Function1/1 -> Bus Creator/1  "α"
  MATLAB Function/1(module) -> Mux1/2, Bus Creator/3  "V"
  controllo divisione per 0 su alpha/1(y) -> Trigonometric Function1/1
  controllo divisione per 0 su beta/1(y) -> Trigonometric Function2/1
  Trigonometric Function2/1 -> Bus Creator/2  "β"
  Vb/1 -> MATLAB Function1/1(V), Switch/2, Switch1/2, Sum2/2  "Va"
  Sum2/1 -> "V effettiva "/1, Demux7/1, MATLAB Function/1(V)  "Va"
  Mux/1 -> controllo divisione per 0 su alpha/1(u)
  Demux7/3 -> Mux/1  "wa"
  Demux7/1 -> Mux/2  "ua"
  Mux1/1 -> controllo divisione per 0 su beta/1(u)
  Demux7/2 -> Mux1/1  "va"
  Constant Wind/1 -> Product/2  "Vw"
  h/1 -> Dryden Wind Turbulence Model (Continuous (-q +r))/1, Wind Shear Model/1
  LBE/1 -> Product/1, Dryden Wind Turbulence Model (Continuous (-q +r))/3, Product1/1, Wind Shear Model/2
  Dryden Wind Turbulence Model (Continuous (-q +r))/1 -> Switch/1
  Constant/1 -> Switch/3
  Dryden Wind Turbulence Model (Continuous (-q +r))/2 -> Switch1/1
  Constant1/1 -> Switch1/3
  Wind Shear Model/1 -> Sum/1
  Product1/1 -> Sum/2
  Switch/1 -> Sum/3
  Switch1/1 -> Terminator/1
  Product/1 -> Sum/4
  Sum/1 -> Scope/1, Sum2/1  "Vento complessivo in B"
  MATLAB Function1/1(module) -> Dryden Wind Turbulence Model (Continuous (-q +r))/2, Discrete Wind Gust Model/1
  Discrete Wind Gust Model/1 -> Product1/2

== system v2022_Modello_SITL_AENEA_2020b/AENEA /AENEA II_SITL1/Weight ==
  LBE : Inport
  Vect_Costanti : Inport  Port=2
  Bus Selector : BusSelector  OutputSignals=Coef_Geometrici.W
  Display1 : Display
  Display3 : Display
  Product3 : Product  Multiplication=Matrix(*)
  "Forzapeso " : Outport  VectorParamsAs1DForOutWhenUnconnected=off
  wires:
  Product3/1 -> "Forzapeso "/1, Display3/1
  LBE/1 -> Product3/1
  Vect_Costanti/1 -> Bus Selector/1
  Bus Selector/1 -> Display1/1, Product3/2  "<W>"

== system v2022_Modello_SITL_AENEA_2020b/AENEA /toSensors/Calc_GS ==
  In1 : Inport
  Add : Sum
  Demux : Demux  Outputs=3
  Sqrt : Sqrt  SaturateOnIntegerOverflow=on
  Square1 : Math  Operator=square  SignedPower=on  SaturateOnIntegerOverflow=on
  Square2 : Math  Operator=square  SignedPower=on  SaturateOnIntegerOverflow=on
  Terminator : Terminator
  GS : Outport  VectorParamsAs1DForOutWhenUnconnected=off
  wires:
  In1/1 -> Demux/1
  Demux/2 -> Square1/1
  Demux/1 -> Square2/1
  Demux/3 -> Terminator/1
  Square2/1 -> Add/1
  Square1/1 -> Add/2
  Add/1 -> Sqrt/1
  Sqrt/1 -> GS/1

== system v2022_Modello_SITL_AENEA_2020b/AENEA /toSensors/Calc_heading ==
  In1 : Inport
  Atan2 : Trigonometry  Operator=atan2
  Demux : Demux  Outputs=3
  Scope : Scope
  Terminator : Terminator
  Heading : Outport  VectorParamsAs1DForOutWhenUnconnected=off
  wires:
  In1/1 -> Demux/1
  Demux/3 -> Terminator/1
  Demux/2 -> Atan2/1
  Demux/1 -> Atan2/2
  Atan2/1 -> Scope/1, Heading/1

== system v2022_Modello_SITL_AENEA_2020b/AENEA /toSensors/To_Lat_Long_MSL ==
  note: Navigation equation
  note: Position derivatives
  V_NED : Inport
  Demux1 : Demux  Outputs=3
      settings: DisplayOption=none
  Demux3 : Demux  Outputs=3
      settings: DisplayOption=none
  Gain : Gain  Gain=-1
  Latitude Bound : Subsystem  mask(Latitude bound){}
      mask help: Bounds the latitude to [-pi/2, pi/2]. When the lower bound is exceeded the latitude is increasing again; when the upper bound is exceeded the latitude is decreasing.
  Longitude Bound : Subsystem  mask(Longitude bound){}
      mask help: Bounds the longitude to [-pi, pi]. When -pi bound is exceeded the longitude wraps back to pi; when the pi bound is exceeded the longitude wraps back to -pi.
  Mux : Mux  Inputs=3
  Mux1 : Mux  Inputs=3
  Position Integrator2 : Integrator  InitialCondition=[latitudineINI longitudineINI HINI]
  Radius at Geocentric Latitude : aerolibasang/Radius at Geocentric Latitude  units=Metric (MKS)  ptype=Earth (WGS84)  F=1/298.257223563  R=6378137
      settings: SourceProductBaseCode=AE
  Sum : Sum  Inputs=|++  InputSameDT=on  SaturateOnIntegerOverflow=on  OutDataTypeStr=Inherit: Same as first input
  Sum1 : Sum  Inputs=|++  InputSameDT=on  SaturateOnIntegerOverflow=on  OutDataTypeStr=Inherit: Same as first input
  Ve/(Rn+h)cos(phi) : Product  Inputs=*//  InputSameDT=on  SaturateOnIntegerOverflow=on  OutDataTypeStr=Inherit: Same as first input
  Vn/(Rm+h) : Product  Inputs=*/  InputSameDT=on  SaturateOnIntegerOverflow=on  OutDataTypeStr=Inherit: Same as first input
  cos(phi) : Trigonometry  Operator=cos
  Position : Outport  VectorParamsAs1DForOutWhenUnconnected=off
  wires:
  Latitude Bound/1(Out) -> cos(phi)/1, Radius at Geocentric Latitude/1, Mux1/1  "lat_optim"
  Longitude Bound/1(Out) -> Mux1/2
  cos(phi)/1 -> Ve/(Rn+h)cos(phi)/3
  Sum1/1 -> Ve/(Rn+h)cos(phi)/2
  Demux3/1 -> Latitude Bound/1(In)
  Ve/(Rn+h)cos(phi)/1 -> Mux/2
  Demux3/2 -> Longitude Bound/1(In)
  Mux1/1 -> Position/1
  Position Integrator2/1 -> Demux3/1
  Demux1/2 -> Ve/(Rn+h)cos(phi)/1
  Mux/1 -> Position Integrator2/1
  Sum/1 -> Vn/(Rm+h)/2
  V_NED/1 -> Demux1/1
  Vn/(Rm+h)/1 -> Mux/1
  Demux3/3 -> Sum/2, Sum1/2, Mux1/3
  Demux1/1 -> Vn/(Rm+h)/1
  Gain/1 -> Mux/3
  Demux1/3 -> Gain/1
  Radius at Geocentric Latitude/1 -> Sum1/1, Sum/1

== system v2022_Modello_SITL_AENEA_2020b/Ricezione segnali2/Subsystem1/AILERON ==
  In1 : Inport
  Constant : Constant  Value=167
  Gain : Gain  Gain=1/9
  Sum : Sum  Inputs=|+-
  Out1 : Outport  VectorParamsAs1DForOutWhenUnconnected=off
  wires:
  Gain/1 -> Sum/1
  Constant/1 -> Sum/2
  Sum/1 -> Out1/1
  In1/1 -> Gain/1

== system v2022_Modello_SITL_AENEA_2020b/Ricezione segnali2/Subsystem1/ELEVATOR ==
  In1 : Inport
  Constant : Constant  Value=75175/447
  Gain : Gain  Gain=50/447
  Sum : Sum  Inputs=|+-
  Out1 : Outport  VectorParamsAs1DForOutWhenUnconnected=off
  wires:
  In1/1 -> Gain/1
  Constant/1 -> Sum/2
  Sum/1 -> Out1/1
  Gain/1 -> Sum/1

== system v2022_Modello_SITL_AENEA_2020b/Ricezione segnali2/Subsystem1/RUDDER ==
  In1 : Inport
  Constant : Constant  Value=75175/447
  Gain : Gain  Gain=50/447
  Sum : Sum  Inputs=|+-
  Out1 : Outport  VectorParamsAs1DForOutWhenUnconnected=off
  wires:
  Gain/1 -> Sum/1
  Constant/1 -> Sum/2
  Sum/1 -> Out1/1
  In1/1 -> Gain/1

== system v2022_Modello_SITL_AENEA_2020b/Ricezione segnali2/Subsystem1/THROTTLE ==
  In1 : Inport
  Constant : Constant  Value=11/8
  Constant2 : Constant  Value=0
  Gain : Gain  Gain=1/800
  Sum : Sum  Inputs=|+-
  Switch : Switch  Criteria=u2 > Threshold  Threshold=0.003
  Out1 : Outport  VectorParamsAs1DForOutWhenUnconnected=off
  wires:
  In1/1 -> Gain/1
  Constant/1 -> Sum/2
  Gain/1 -> Sum/1
  Switch/1 -> Out1/1
  Sum/1 -> Switch/1, Switch/2
  Constant2/1 -> Switch/3

== system v2022_Modello_SITL_AENEA_2020b/Sensori/GPS1/Latitudine e Longitudine ==
  lat : Inport
  long : Inport  Port=2
  C/Long1 : Constant  Value=Std_con_long
  C/lat : Constant  Value=Std_con_lat
  Gain : Gain  Gain=1/Ta_lat  SaturateOnIntegerOverflow=on  OutDataTypeStr=Inherit: Same as input  ParamDataTypeStr=Inherit: Same as input
  Gain1 : Gain  Gain=1/Ta_long  SaturateOnIntegerOverflow=on  OutDataTypeStr=Inherit: Same as input  ParamDataTypeStr=Inherit: Same as input
  Integrator : Integrator
  Integrator1 : Integrator
  Multiply{,1..3} (4 alike) : Product
  Sum : Sum  Inputs=|+-  InputSameDT=on  SaturateOnIntegerOverflow=on  OutDataTypeStr=Inherit: Same as first input
  Sum1 : Sum  Inputs=|++  InputSameDT=on  SaturateOnIntegerOverflow=on  OutDataTypeStr=Inherit: Same as first input
  Sum2 : Sum  Inputs=|+-  InputSameDT=on  SaturateOnIntegerOverflow=on  OutDataTypeStr=Inherit: Same as first input
  Sum3 : Sum  Inputs=|++  InputSameDT=on  SaturateOnIntegerOverflow=on  OutDataTypeStr=Inherit: Same as first input
  To Workspace : ToWorkspace  Commented=on  VariableName=errore_long1  SampleTime=-1
      settings: Save2DSignal=2-D array (concatenate along first dimension)
  To Workspace1 : ToWorkspace  Commented=on  VariableName=errore_lat1  SampleTime=-1
      settings: Save2DSignal=2-D array (concatenate along first dimension)
  White Noise : RandomNumber  Seed=randi([0 2000],1,1)  SampleTime=Ts_gps
  White Noise2 : RandomNumber  Seed=randi([0 2000],1,1)  SampleTime=Ts_gps
  Latitudine : Outport
  Longitudine : Outport  Port=2
  wires:
  Multiply3/1 -> Multiply2/1
  Multiply1/1 -> Multiply/1
  long/1 -> Multiply1/1, Sum1/1
  White Noise2/1 -> Multiply/2
  C/lat/1 -> Multiply3/2
  C/Long1/1 -> Multiply1/2
  Multiply2/1 -> Sum2/1
  lat/1 -> Sum3/1, Multiply3/1
  Multiply/1 -> Sum/1
  Sum1/1 -> Longitudine/1
  Sum2/1 -> Integrator1/1
  Integrator/1 -> Sum1/2, To Workspace/1, Gain1/1
  Gain1/1 -> Sum/2
  Sum/1 -> Integrator/1
  Sum3/1 -> Latitudine/1
  Gain/1 -> Sum2/2
  White Noise/1 -> Multiply2/2
  Integrator1/1 -> Gain/1, Sum3/2, To Workspace1/1

== system v2022_Modello_SITL_AENEA_2020b/Sensori/GPS1/Subsystem ==
  Lat : Inport
  C/Lat1 : Constant  Value=Std_con_lat
  Delay_gps : TransportDelay  DelayTime=delay_gps  InitialOutput=latitudineINI
  Gain : Gain  Gain=1/Ta_lat  SaturateOnIntegerOverflow=on  OutDataTypeStr=Inherit: Same as input  ParamDataTypeStr=Inherit: Same as input
  Integrator : Integrator
  Multiply : Product
  Multiply1 : Product
  Sum : Sum  Inputs=|+-  InputSameDT=on  SaturateOnIntegerOverflow=on  OutDataTypeStr=Inherit: Same as first input
  Sum1 : Sum  Inputs=|++  InputSameDT=on  SaturateOnIntegerOverflow=on  OutDataTypeStr=Inherit: Same as first input
  To Workspace : ToWorkspace  Commented=on  VariableName=errore_lat  SaveFormat=Timeseries  SampleTime=-1
  White Noise : RandomNumber  Seed=seed_gps  SampleTime=Ts_gps
  Out1 : Outport  VectorParamsAs1DForOutWhenUnconnected=off
  wires:
  Sum1/1 -> Out1/1
  Integrator/1 -> Gain/1, Sum1/2, To Workspace/1
  Sum/1 -> Integrator/1
  Delay_gps/1 -> Multiply1/1, Sum1/1
  Gain/1 -> Sum/2
  White Noise/1 -> Multiply/2
  Multiply/1 -> Sum/1
  Lat/1 -> Delay_gps/1
  C/Lat1/1 -> Multiply1/2
  Multiply1/1 -> Multiply/1

== system v2022_Modello_SITL_AENEA_2020b/Sensori/GPS1/Subsystem1 ==
  Long : Inport
  C/Long1 : Constant  Value=Std_con_long
  Delay_gps : TransportDelay  DelayTime=delay_gps  InitialOutput=longitudineINI
  Gain1 : Gain  Gain=1/Ta_long  SaturateOnIntegerOverflow=on  OutDataTypeStr=Inherit: Same as input  ParamDataTypeStr=Inherit: Same as input
  Integrator : Integrator
  Multiply : Product
  Multiply1 : Product
  Sum : Sum  Inputs=|+-  InputSameDT=on  SaturateOnIntegerOverflow=on  OutDataTypeStr=Inherit: Same as first input
  Sum1 : Sum  Inputs=|++  InputSameDT=on  SaturateOnIntegerOverflow=on  OutDataTypeStr=Inherit: Same as first input
  To Workspace : ToWorkspace  VariableName=errore_long  SaveFormat=Timeseries  SampleTime=-1
  White Noise : RandomNumber  Seed=seed_gps  SampleTime=Ts_gps
  long_out : Outport  VectorParamsAs1DForOutWhenUnconnected=off
  wires:
  Multiply/1 -> Sum/1
  White Noise/1 -> Multiply/2
  Gain1/1 -> Sum/2
  Sum1/1 -> long_out/1
  Delay_gps/1 -> Multiply1/1, Sum1/1
  Sum/1 -> Integrator/1
  Integrator/1 -> Sum1/2, To Workspace/1, Gain1/1
  Multiply1/1 -> Multiply/1
  C/Long1/1 -> Multiply1/2
  Long/1 -> Delay_gps/1

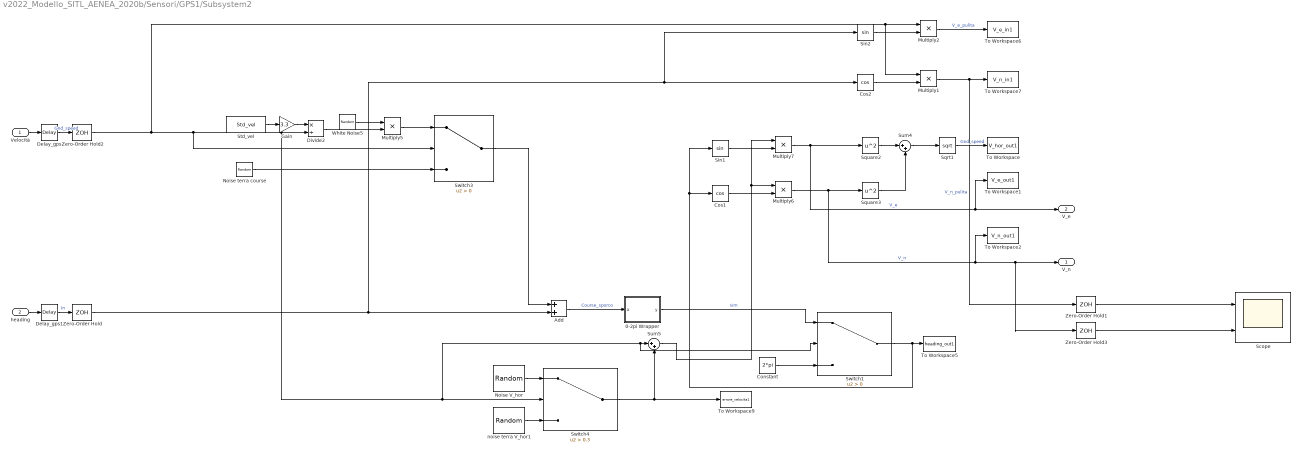
== system v2022_Modello_SITL_AENEA_2020b/Sensori/GPS1/Subsystem2 ==
  Velocità : Inport
  heading : Inport  Port=2
  0-2pi Wrapper : MATLAB Function  TreatAsAtomicUnit=on
  Add : Sum
  Constant : Constant  Value=2*pi
  Cos1 : Trigonometry  Operator=cos
  Cos2 : Trigonometry  Operator=cos
  Delay_gps : TransportDelay  DelayTime=delay_gps  InitialOutput=V_cruise
  Delay_gps1 : TransportDelay  DelayTime=delay_gps
  Divide2 : Product  Inputs=*/
  Gain : Gain  Gain=3.3
  Multiply{1..2,5..7} (5 alike) : Product
  Noise V_hor : RandomNumber  Variance=Std_vel^2  Seed=seed_gps  SampleTime=Ts_gps
  Noise terra course : RandomNumber  Variance=Var_heading_static  Seed=seed_gps  SampleTime=0.02
  Scope : Scope  NumInputPorts=2
  Sin1 : Trigonometry
  Sin2 : Trigonometry
  Sqrt1 : Sqrt  SaturateOnIntegerOverflow=on
  Square2 : Math  Operator=square  SignedPower=on  SaturateOnIntegerOverflow=on
  Square3 : Math  Operator=square  SignedPower=on  SaturateOnIntegerOverflow=on
  Std_vel : Constant  Value=Std_vel
  Sum4 : Sum  Inputs=|++
  Sum5 : Sum  Inputs=|++
  Switch1 : Switch  Criteria=u2 > Threshold
  Switch3 : Switch  Criteria=u2 > Threshold
  Switch4 : Switch  Criteria=u2 > Threshold  Threshold=0.3
  To Workspace : ToWorkspace  VariableName=V_hor_out1  SaveFormat=Timeseries  SampleTime=-1
  To Workspace1 : ToWorkspace  VariableName=V_e_out1  SaveFormat=Timeseries  SampleTime=-1
  To Workspace2 : ToWorkspace  VariableName=V_n_out1  SaveFormat=Timeseries  SampleTime=-1
  To Workspace5 : ToWorkspace  VariableName=heading_out1  SaveFormat=Timeseries  SampleTime=-1
  To Workspace6 : ToWorkspace  VariableName=V_e_in1  SaveFormat=Timeseries  SampleTime=-1
  To Workspace7 : ToWorkspace  VariableName=V_n_in1  SaveFormat=Timeseries  SampleTime=-1
  To Workspace9 : ToWorkspace  VariableName=errore_velocita1  SaveFormat=Timeseries  SampleTime=-1
  White Noise5 : RandomNumber  Variance=0.1  Seed=seed_gps  SampleTime=0.02
  Zero-Order Hold : ZeroOrderHold  SampleTime=0.02
  Zero-Order Hold1 : ZeroOrderHold  SampleTime=0.2
  Zero-Order Hold2 : ZeroOrderHold  SampleTime=0.02
  Zero-Order Hold3 : ZeroOrderHold  SampleTime=0.2
  noise terra V_hor1 : RandomNumber  Variance=Var_V_hor_static  Seed=seed_gps  SampleTime=Ts_gps
  "V_n " : Outport  VectorParamsAs1DForOutWhenUnconnected=off
  V_e : Outport  Port=2  VectorParamsAs1DForOutWhenUnconnected=off
  wires:
  Zero-Order Hold2/1 -> Multiply2/1, Multiply1/1, Switch3/2, Divide2/2, Switch4/2, Sum5/1, Switch1/2
  Zero-Order Hold/1 -> Add/2, Sin2/1, Cos2/1
  Switch1/1 -> To Workspace5/1, Cos1/1, Sin1/1
  Constant/1 -> Switch1/3
  Sqrt1/1 -> To Workspace/1  "Gnd_speed"
  Divide2/1 -> Multiply5/2
  Velocità/1 -> Delay_gps/1
  heading/1 -> Delay_gps1/1
  Sin2/1 -> Multiply2/2
  Sin1/1 -> Multiply7/2
  Noise terra course/1 -> Switch3/3
  0-2pi Wrapper/1(y) -> Switch1/1  "sim"
  Cos2/1 -> Multiply1/2
  Multiply2/1 -> To Workspace6/1  "V_e_pulita"
  Multiply1/1 -> Zero-Order Hold1/1, To Workspace7/1  "V_n_pulita"
  Noise V_hor/1 -> Switch4/1
  Switch3/1 -> Add/1
  Cos1/1 -> Multiply6/2
  Sum4/1 -> Sqrt1/1
  Multiply7/1 -> Square2/1, V_e/1, To Workspace1/1  "V_e"
  White Noise5/1 -> Multiply5/1
  Delay_gps/1 -> Zero-Order Hold2/1  "Gnd_speed"
  Sum5/1 -> Multiply7/1, Multiply6/1
  Multiply6/1 -> Square3/1, To Workspace2/1, Zero-Order Hold3/1, "V_n "/1  "V_n"
  Square2/1 -> Sum4/1
  Multiply5/1 -> Switch3/1
  Add/1 -> 0-2pi Wrapper/1(a)  "Course_sporco"
  Delay_gps1/1 -> Zero-Order Hold/1  "In"
  Square3/1 -> Sum4/2
  noise terra V_hor1/1 -> Switch4/3
  Switch4/1 -> Sum5/2, To Workspace9/1
  Zero-Order Hold1/1 -> Scope/1
  Zero-Order Hold3/1 -> Scope/2
  Std_vel/1 -> Gain/1
  Gain/1 -> Divide2/1

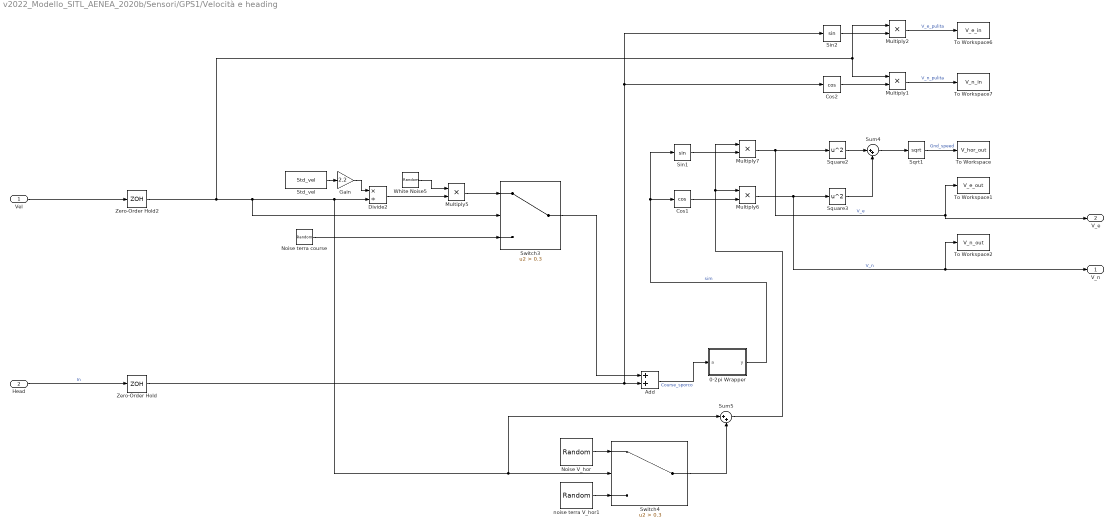
== system v2022_Modello_SITL_AENEA_2020b/Sensori/GPS1/Velocità e heading ==
  Vel : Inport
  Head : Inport  Port=2
  0-2pi Wrapper : MATLAB Function  TreatAsAtomicUnit=on
  Add : Sum
  Cos1 : Trigonometry  Operator=cos
  Cos2 : Trigonometry  Operator=cos
  Divide2 : Product  Inputs=*/
  Gain : Gain  Gain=2.2
  Multiply{1..2,5..7} (5 alike) : Product
  Noise V_hor : RandomNumber  Variance=Var_heading  Seed=randi([0 2000],1,1)  SampleTime=Ts_gps
  Noise terra course : RandomNumber  Variance=Var_V_hor_static  Seed=randi([0 2000],1,1)  SampleTime=Ts_gps
  Sin1 : Trigonometry
  Sin2 : Trigonometry
  Sqrt1 : Sqrt  SaturateOnIntegerOverflow=on
  Square2 : Math  Operator=square  SignedPower=on  SaturateOnIntegerOverflow=on
  Square3 : Math  Operator=square  SignedPower=on  SaturateOnIntegerOverflow=on
  Std_vel : Constant  Value=Std_vel  SampleTime=Ts_gps
  Sum4 : Sum  Inputs=|++
  Sum5 : Sum  Inputs=|++
  Switch3 : Switch  Criteria=u2 > Threshold  Threshold=0.3
  Switch4 : Switch  Criteria=u2 > Threshold  Threshold=0.3
  To Workspace : ToWorkspace  VariableName=V_hor_out  SaveFormat=Timeseries  SampleTime=-1
  To Workspace1 : ToWorkspace  VariableName=V_e_out  SaveFormat=Timeseries  SampleTime=-1
  To Workspace2 : ToWorkspace  VariableName=V_n_out  SaveFormat=Timeseries  SampleTime=-1
  To Workspace6 : ToWorkspace  VariableName=V_e_in  SaveFormat=Timeseries  SampleTime=-1
  To Workspace7 : ToWorkspace  VariableName=V_n_in  SaveFormat=Timeseries  SampleTime=-1
  White Noise5 : RandomNumber  Variance=Var_V_hor  Seed=randi([0 2000],1,1)  SampleTime=Ts_gps
  Zero-Order Hold : ZeroOrderHold  SampleTime=0.02
  Zero-Order Hold2 : ZeroOrderHold  SampleTime=0.02
  noise terra V_hor1 : RandomNumber  Variance=Var_heading_static  Seed=randi([0 2000],1,1)  SampleTime=Ts_gps
  "V_n " : Outport  VectorParamsAs1DForOutWhenUnconnected=off
  V_e : Outport  Port=2  VectorParamsAs1DForOutWhenUnconnected=off
  wires:
  Gain/1 -> Divide2/1
  Noise terra course/1 -> Switch3/3
  Divide2/1 -> Multiply5/2
  Std_vel/1 -> Gain/1
  Multiply5/1 -> Switch3/1
  Head/1 -> Zero-Order Hold/1  "In"
  Switch4/1 -> Sum5/2
  White Noise5/1 -> Multiply5/1
  0-2pi Wrapper/1(y) -> Cos1/1, Sin1/1  "sim"
  Switch3/1 -> Add/1
  Noise V_hor/1 -> Switch4/1
  Vel/1 -> Zero-Order Hold2/1
  noise terra V_hor1/1 -> Switch4/3
  Add/1 -> 0-2pi Wrapper/1(a)  "Course_sporco"
  Cos1/1 -> Multiply6/2
  Multiply7/1 -> Square2/1, V_e/1, To Workspace1/1  "V_e"
  Multiply1/1 -> To Workspace7/1  "V_n_pulita"
  Cos2/1 -> Multiply1/2
  Zero-Order Hold/1 -> Sin2/1, Cos2/1, Add/2
  Zero-Order Hold2/1 -> Multiply2/1, Multiply1/1, Divide2/2, Switch4/2, Sum5/1, Switch3/2
  Sqrt1/1 -> To Workspace/1  "Gnd_speed"
  Sin2/1 -> Multiply2/2
  Sum4/1 -> Sqrt1/1
  Multiply6/1 -> Square3/1, To Workspace2/1, "V_n "/1  "V_n"
  Square3/1 -> Sum4/2
  Square2/1 -> Sum4/1
  Sum5/1 -> Multiply7/1, Multiply6/1
  Sin1/1 -> Multiply7/2
  Multiply2/1 -> To Workspace6/1  "V_e_pulita"

== system v2022_Modello_SITL_AENEA_2020b/Sensori/int1/INT16  ==
  <u> : Inport
  Data Type Conversion : DataTypeConversion  OutDataTypeStr=int16  LockScale=on
  Data Type Conversion1 : DataTypeConversion  OutDataTypeStr=double  LockScale=on
  Gain : Gain  Gain=100
  Gain1 : Gain  Gain=1/100
  Out1 : Outport  VectorParamsAs1DForOutWhenUnconnected=off
  wires:
  <u>/1 -> Gain/1
  Gain1/1 -> Out1/1
  Gain/1 -> Data Type Conversion/1
  Data Type Conversion/1 -> Data Type Conversion1/1
  Data Type Conversion1/1 -> Gain1/1

== system v2022_Modello_SITL_AENEA_2020b/Sensori/int16/INT16  ==
  <u> : Inport
  Data Type Conversion : DataTypeConversion  OutDataTypeStr=int16  LockScale=on
  Data Type Conversion1 : DataTypeConversion  OutDataTypeStr=double  LockScale=on
  Gain : Gain  Gain=100
  Gain1 : Gain  Gain=1/100
  Out1 : Outport  VectorParamsAs1DForOutWhenUnconnected=off
  wires:
  Data Type Conversion1/1 -> Gain1/1
  Data Type Conversion/1 -> Data Type Conversion1/1
  Gain/1 -> Data Type Conversion/1
  Gain1/1 -> Out1/1
  <u>/1 -> Gain/1

== system v2022_Modello_SITL_AENEA_2020b/Sensori/int16_rad /INT16  ==
  <u> : Inport
  Data Type Conversion : DataTypeConversion  OutDataTypeStr=int16  LockScale=on
  Data Type Conversion1 : DataTypeConversion  OutDataTypeStr=double  LockScale=on
  Gain : Gain  Gain=100
  Gain1 : Gain  Gain=1/100
  Out1 : Outport  VectorParamsAs1DForOutWhenUnconnected=off
  wires:
  <u>/1 -> Gain/1
  Gain1/1 -> Out1/1
  Gain/1 -> Data Type Conversion/1
  Data Type Conversion/1 -> Data Type Conversion1/1
  Data Type Conversion1/1 -> Gain1/1

== system v2022_Modello_SITL_AENEA_2020b/Sensori/int16_rad 1/INT16  ==
  <u> : Inport
  Data Type Conversion : DataTypeConversion  OutDataTypeStr=int16  LockScale=on
  Data Type Conversion1 : DataTypeConversion  OutDataTypeStr=double  LockScale=on
  Gain : Gain  Gain=100
  Gain1 : Gain  Gain=1/100
  Out1 : Outport  VectorParamsAs1DForOutWhenUnconnected=off
  wires:
  Data Type Conversion1/1 -> Gain1/1
  Data Type Conversion/1 -> Data Type Conversion1/1
  Gain/1 -> Data Type Conversion/1
  Gain1/1 -> Out1/1
  <u>/1 -> Gain/1

== system v2022_Modello_SITL_AENEA_2020b/Sensori/int16_rad 2/INT16  ==
  <u> : Inport
  Data Type Conversion : DataTypeConversion  OutDataTypeStr=int16  LockScale=on
  Data Type Conversion1 : DataTypeConversion  OutDataTypeStr=double  LockScale=on
  Gain : Gain  Gain=100
  Gain1 : Gain  Gain=1/100
  Out1 : Outport  VectorParamsAs1DForOutWhenUnconnected=off
  wires:
  <u>/1 -> Gain/1
  Gain1/1 -> Out1/1
  Gain/1 -> Data Type Conversion/1
  Data Type Conversion/1 -> Data Type Conversion1/1
  Data Type Conversion1/1 -> Gain1/1

== system v2022_Modello_SITL_AENEA_2020b/Sensori/int16_rad 3/INT16  ==
  <u> : Inport
  Data Type Conversion : DataTypeConversion  OutDataTypeStr=int16  LockScale=on
  Data Type Conversion1 : DataTypeConversion  OutDataTypeStr=double  LockScale=on
  Gain : Gain  Gain=100
  Gain1 : Gain  Gain=1/100
  Out1 : Outport  VectorParamsAs1DForOutWhenUnconnected=off
  wires:
  Data Type Conversion1/1 -> Gain1/1
  Data Type Conversion/1 -> Data Type Conversion1/1
  Gain/1 -> Data Type Conversion/1
  Gain1/1 -> Out1/1
  <u>/1 -> Gain/1

== system v2022_Modello_SITL_AENEA_2020b/Sensori/int16_rad 4/INT16  ==
  <u> : Inport
  Data Type Conversion : DataTypeConversion  OutDataTypeStr=int16  LockScale=on
  Data Type Conversion1 : DataTypeConversion  OutDataTypeStr=double  LockScale=on
  Gain : Gain  Gain=100
  Gain1 : Gain  Gain=1/100
  Out1 : Outport  VectorParamsAs1DForOutWhenUnconnected=off
  wires:
  <u>/1 -> Gain/1
  Gain1/1 -> Out1/1
  Gain/1 -> Data Type Conversion/1
  Data Type Conversion/1 -> Data Type Conversion1/1
  Data Type Conversion1/1 -> Gain1/1

== system v2022_Modello_SITL_AENEA_2020b/Sensori/int16_rad 5/INT16  ==
  <u> : Inport
  Data Type Conversion : DataTypeConversion  OutDataTypeStr=int16  LockScale=on
  Data Type Conversion1 : DataTypeConversion  OutDataTypeStr=double  LockScale=on
  Gain : Gain  Gain=100
  Gain1 : Gain  Gain=1/100
  Out1 : Outport  VectorParamsAs1DForOutWhenUnconnected=off
  wires:
  Data Type Conversion1/1 -> Gain1/1
  Data Type Conversion/1 -> Data Type Conversion1/1
  Gain/1 -> Data Type Conversion/1
  Gain1/1 -> Out1/1
  <u>/1 -> Gain/1

== system v2022_Modello_SITL_AENEA_2020b/Sensori/int2/INT16  ==
  <u> : Inport
  Data Type Conversion : DataTypeConversion  OutDataTypeStr=int16  LockScale=on
  Data Type Conversion1 : DataTypeConversion  OutDataTypeStr=double  LockScale=on
  Gain : Gain  Gain=100
  Gain1 : Gain  Gain=1/100
  Out1 : Outport  VectorParamsAs1DForOutWhenUnconnected=off
  wires:
  Data Type Conversion1/1 -> Gain1/1
  Data Type Conversion/1 -> Data Type Conversion1/1
  Gain/1 -> Data Type Conversion/1
  Gain1/1 -> Out1/1
  <u>/1 -> Gain/1
